simulink model "EC_bloqueo_sobreescritura"  (R2023b)
settings: Solver=VariableStepAuto  StartTime=0.0  StopTime=20  RelTol=1e-3
settings Model: Creator=anruk  LastModifiedBy=anruk

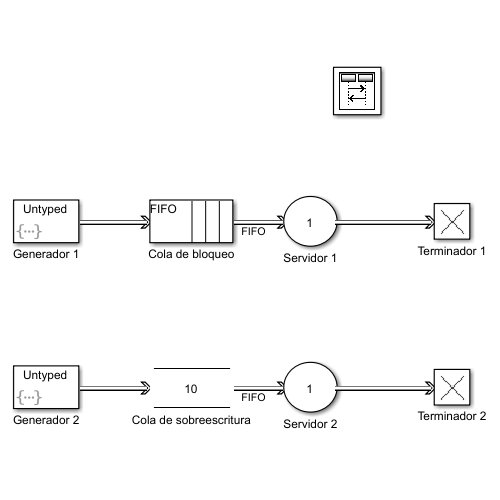
[thumbnail: Simulink's stored preview of the top-level diagram]
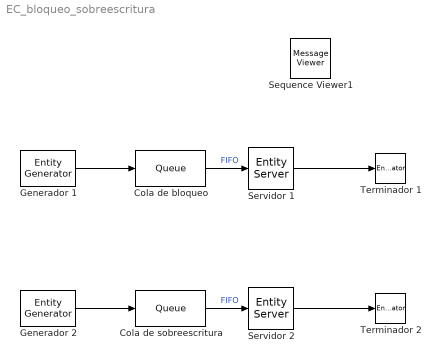
== system EC_bloqueo_sobreescritura ==
  Cola de bloqueo : Queue  InputPortMessageModes=m  OutputPortMessageModes=m  Capacity=10
  Cola de sobreescritura : Queue  InputPortMessageModes=m  OutputPortMessageModes=m  OverwriteOldest=on  Capacity=10
  Generador 1 : EntityGenerator  OutputPortMessageModes=m  GenerateAction=entity = rand();  AttributeName=entity  AttributeInitialValue=0  EntityTypeName=Entity
  Generador 2 : EntityGenerator  OutputPortMessageModes=m  GenerateAction=entity=rand();  AttributeName=entity  AttributeInitialValue=0  EntityTypeName=Entity
  Sequence Viewer1 : MessageViewer  History=1000  SavedRootId=#
  Servidor 1 : EntityServer  InputPortMessageModes=m  OutputPortMessageModes=m  Capacity=1  ServiceTimeValue=25
  Servidor 2 : EntityServer  InputPortMessageModes=m  OutputPortMessageModes=m  Capacity=1  ServiceTimeValue=25
  Terminador 1 : EntityTerminator  InputPortMessageModes=m
  Terminador 2 : EntityTerminator  InputPortMessageModes=m
  wires:
  Generador 1/1 -> Cola de bloqueo/1
  Cola de bloqueo/1 -> Servidor 1/1  "FIFO"
  Generador 2/1 -> Cola de sobreescritura/1
  Servidor 2/1 -> Terminador 2/1
  Cola de sobreescritura/1 -> Servidor 2/1  "FIFO"
  Servidor 1/1 -> Terminador 1/1
